simulink library "mylib"  (R2019b)
settings: Solver=VariableStepAuto  StartTime=0.0  StopTime=10.0  RelTol=1e-3
undefined symbols (not defined in the file or in its folder): AG, AH, AV, BCHL, BCHV, BG, BH, CG, CH, magnitude, Ts, XMW
libraries: $bdroot x28, TElib x2
(part 3 of 3)

== system mylib/Process Noise I=1-12 G New/TESUB6/Subsystem/TESUB7(3) ==
  G : Inport
  I : Constant  Value=3
  TESUB7 : $bdroot/TESUB7 G-New  SystemSampleTime=-1  Latency=0  AutoFrameSizeCalculation=off
  TESUB7(3) : Outport  VectorParamsAs1DForOutWhenUnconnected=off
  G_NEW : Outport  Port=2  VectorParamsAs1DForOutWhenUnconnected=off
  wires:
  I/1 -> TESUB7/1
  TESUB7/2 -> G_NEW/1
  G/1 -> TESUB7/2
  TESUB7/1 -> TESUB7(3)/1

== system mylib/Process Noise I=1-12 G New/TESUB6/Subsystem/TESUB7(4) ==
  G : Inport
  I : Constant  Value=4
  TESUB7 : $bdroot/TESUB7 G-New  SystemSampleTime=-1  Latency=0  AutoFrameSizeCalculation=off
  TESUB7(4) : Outport  VectorParamsAs1DForOutWhenUnconnected=off
  G_NEW : Outport  Port=2  VectorParamsAs1DForOutWhenUnconnected=off
  wires:
  I/1 -> TESUB7/1
  TESUB7/2 -> G_NEW/1
  G/1 -> TESUB7/2
  TESUB7/1 -> TESUB7(4)/1

== system mylib/Process Noise I=1-12 G New/TESUB6/Subsystem/TESUB7(5) ==
  G : Inport
  I : Constant  Value=5
  TESUB7 : $bdroot/TESUB7 G-New  SystemSampleTime=-1  Latency=0  AutoFrameSizeCalculation=off
  TESUB7(5) : Outport  VectorParamsAs1DForOutWhenUnconnected=off
  G_NEW : Outport  Port=2  VectorParamsAs1DForOutWhenUnconnected=off
  wires:
  I/1 -> TESUB7/1
  TESUB7/2 -> G_NEW/1
  G/1 -> TESUB7/2
  TESUB7/1 -> TESUB7(5)/1

== system mylib/Process Noise I=1-12 G New/TESUB6/Subsystem/TESUB7(6) ==
  G : Inport
  I : Constant  Value=6
  TESUB7 : $bdroot/TESUB7 G-New  SystemSampleTime=-1  Latency=0  AutoFrameSizeCalculation=off
  TESUB7(6) : Outport  VectorParamsAs1DForOutWhenUnconnected=off
  G_NEW : Outport  Port=2  VectorParamsAs1DForOutWhenUnconnected=off
  wires:
  I/1 -> TESUB7/1
  TESUB7/2 -> G_NEW/1
  G/1 -> TESUB7/2
  TESUB7/1 -> TESUB7(6)/1

== system mylib/Process Noise I=1-12 G New/TESUB6/Subsystem/TESUB7(7) ==
  G : Inport
  I : Constant  Value=7
  TESUB7 : $bdroot/TESUB7 G-New  SystemSampleTime=-1  Latency=0  AutoFrameSizeCalculation=off
  TESUB7(7) : Outport  VectorParamsAs1DForOutWhenUnconnected=off
  G_NEW : Outport  Port=2  VectorParamsAs1DForOutWhenUnconnected=off
  wires:
  I/1 -> TESUB7/1
  TESUB7/2 -> G_NEW/1
  G/1 -> TESUB7/2
  TESUB7/1 -> TESUB7(7)/1

== system mylib/Process Noise I=1-12 G New/TESUB6/Subsystem/TESUB7(8) ==
  G : Inport
  I : Constant  Value=8
  TESUB7 : $bdroot/TESUB7 G-New  SystemSampleTime=-1  Latency=0  AutoFrameSizeCalculation=off
  TESUB7(8) : Outport  VectorParamsAs1DForOutWhenUnconnected=off
  G_NEW : Outport  Port=2  VectorParamsAs1DForOutWhenUnconnected=off
  wires:
  I/1 -> TESUB7/1
  TESUB7/2 -> G_NEW/1
  G/1 -> TESUB7/2
  TESUB7/1 -> TESUB7(8)/1

== system mylib/Process Noise I=1-12 G New/TESUB6/Subsystem/TESUB7(9) ==
  G : Inport
  I : Constant  Value=9
  TESUB7 : $bdroot/TESUB7 G-New  SystemSampleTime=-1  Latency=0  AutoFrameSizeCalculation=off
  TESUB7(9) : Outport  VectorParamsAs1DForOutWhenUnconnected=off
  G_NEW : Outport  Port=2  VectorParamsAs1DForOutWhenUnconnected=off
  wires:
  I/1 -> TESUB7/1
  TESUB7/2 -> G_NEW/1
  G/1 -> TESUB7/2
  TESUB7/1 -> TESUB7(9)/1

== system mylib/Process Noise I=23-36/Gas Analysis Delay/Subsystem/If Action Subsystem ==
  Action Port : ActionPort
  Constant : Constant  Value=0
  Out1 : Outport  VectorParamsAs1DForOutWhenUnconnected=off
  wires:
  Constant/1 -> Out1/1

== system mylib/Process Noise I=23-36/Gas Analysis Delay/Subsystem/If Action Subsystem1 ==
  In1 : Inport
  Action Port : ActionPort
  Out1 : Outport  VectorParamsAs1DForOutWhenUnconnected=off
  wires:
  In1/1 -> Out1/1

== system mylib/Process Noise I=37-41/Gas Analysis Delay/Subsystem/If Action Subsystem ==
  Action Port : ActionPort
  Constant : Constant  Value=0
  Out1 : Outport  VectorParamsAs1DForOutWhenUnconnected=off
  wires:
  Constant/1 -> Out1/1

== system mylib/Process Noise I=37-41/Gas Analysis Delay/Subsystem/If Action Subsystem1 ==
  In1 : Inport
  Action Port : ActionPort
  Out1 : Outport  VectorParamsAs1DForOutWhenUnconnected=off
  wires:
  In1/1 -> Out1/1

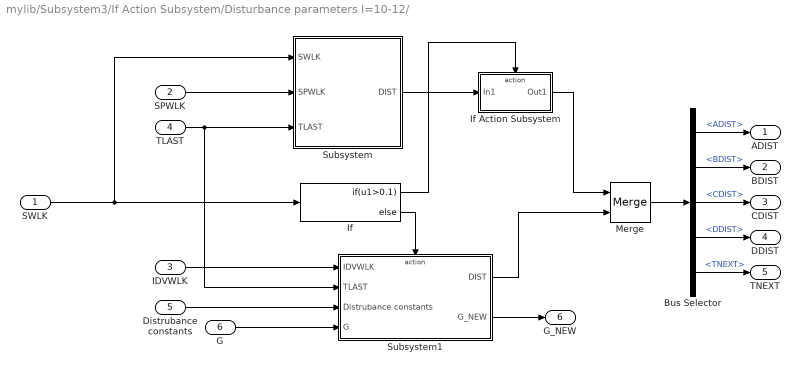
== system mylib/Subsystem3/If Action Subsystem/Disturbance parameters I=10-12/  ==
  SWLK : Inport
  SPWLK : Inport  Port=2
  IDVWLK : Inport  Port=3
  TLAST : Inport  Port=4
  Distrubance constants : Inport  Port=5
  G : Inport  Port=6
  Bus Selector : BusSelector  OutputSignals=ADIST,BDIST,CDIST,DDIST,TNEXT
  If : If  IfExpression=u1>0.1
  If Action Subsystem : Subsystem  TreatAsAtomicUnit=on
  Merge : Merge
  Subsystem : Subsystem
  Subsystem1 : Subsystem
  ADIST : Outport  VectorParamsAs1DForOutWhenUnconnected=off
  BDIST : Outport  Port=2  VectorParamsAs1DForOutWhenUnconnected=off
  CDIST : Outport  Port=3  VectorParamsAs1DForOutWhenUnconnected=off
  DDIST : Outport  Port=4  VectorParamsAs1DForOutWhenUnconnected=off
  TNEXT : Outport  Port=5  VectorParamsAs1DForOutWhenUnconnected=off
  G_NEW : Outport  Port=6  VectorParamsAs1DForOutWhenUnconnected=off
  wires:
  G/1 -> Subsystem1/4(G)
  Bus Selector/5 -> TNEXT/1  "<TNEXT>"
  Bus Selector/4 -> DDIST/1  "<DDIST>"
  Bus Selector/3 -> CDIST/1  "<CDIST>"
  Bus Selector/2 -> BDIST/1  "<BDIST>"
  Bus Selector/1 -> ADIST/1  "<ADIST>"
  Distrubance constants/1 -> Subsystem1/3(Distrubance constants)
  Merge/1 -> Bus Selector/1
  Subsystem1/1(DIST) -> Merge/2
  If Action Subsystem/1(Out1) -> Merge/1
  Subsystem/1(DIST) -> If Action Subsystem/1(In1)
  If/2 -> Subsystem1/Action
  If/1 -> If Action Subsystem/Action
  TLAST/1 -> Subsystem/3(TLAST), Subsystem1/2(TLAST)
  SWLK/1 -> If/1, Subsystem/1(SWLK)
  SPWLK/1 -> Subsystem/2(SPWLK)
  IDVWLK/1 -> Subsystem1/1(IDVWLK)
  Subsystem1/2(G_NEW) -> G_NEW/1

== system mylib/Subsystem3/If Action Subsystem/Disturbance parameters I=10-12/Subsystem ==
  TNEXT : Inport
  TLAST : Inport  Port=2
  HWLK : Sum  Inputs=+-
  "HWLK " : Outport  VectorParamsAs1DForOutWhenUnconnected=off
  wires:
  HWLK/1 -> "HWLK "/1
  TLAST/1 -> HWLK/2
  TNEXT/1 -> HWLK/1

== system mylib/Subsystem3/If Action Subsystem/Disturbance parameters I=10-12/Subsystem1 ==
  ADIST : Inport
  BDIST : Inport  Port=2
  CDIST : Inport  Port=3
  DDIST : Inport  Port=4
  HWLK : Inport  Port=5
  Add : Sum
  Add1 : Sum
  Product : Product
  Product1 : Product
  Product2 : Product
  SWLK : Sum
  "SWLK " : Outport  VectorParamsAs1DForOutWhenUnconnected=off
  wires:
  HWLK/1 -> Product/1, Product1/1, Product2/1
  Add1/1 -> Product2/2
  Product1/1 -> Add1/1
  DDIST/1 -> Product/2
  Product2/1 -> SWLK/2
  Add/1 -> Product1/2
  Product/1 -> Add/1
  SWLK/1 -> "SWLK "/1
  CDIST/1 -> Add/2
  ADIST/1 -> SWLK/1
  BDIST/1 -> Add1/2

== system mylib/Subsystem3/If Action Subsystem/Disturbance parameters I=10-12/Subsystem2 ==
  BDIST : Inport
  CDIST : Inport  Port=2
  DDIST : Inport  Port=3
  HWLK : Inport  Port=4
  Add2 : Sum
  Constant : Constant  Value=3
  Constant1 : Constant  Value=2
  Product3 : Product  Inputs=3
  Product4 : Product
  Product5 : Product
  SPWLK : Sum
  "SPWLK " : Outport  VectorParamsAs1DForOutWhenUnconnected=off
  wires:
  BDIST/1 -> SPWLK/1
  CDIST/1 -> Product4/2
  Constant1/1 -> Product4/1
  Product3/1 -> Add2/1
  HWLK/1 -> Product3/2, Product5/1
  Product5/1 -> SPWLK/2
  Constant/1 -> Product3/1
  Add2/1 -> Product5/2
  SPWLK/1 -> "SPWLK "/1
  Product4/1 -> Add2/2
  DDIST/1 -> Product3/3

== system mylib/Disturbance calculations I=1-9/If Action Subsystem/Disturbance parameters I=1-9/TESUB5/Subsystem ==
  G : Inport
  HSPAN : Inport  Port=2
  HZERO : Inport  Port=3
  Constant : Constant  Value=-1
  H : Sum
  Product : Product
  TESUB7 G-New : $bdroot/TESUB7 G-New  SystemSampleTime=-1  Latency=0  AutoFrameSizeCalculation=off
  "H " : Outport  VectorParamsAs1DForOutWhenUnconnected=off
  G_NEW : Outport  Port=2  VectorParamsAs1DForOutWhenUnconnected=off
  wires:
  HZERO/1 -> H/2
  HSPAN/1 -> Product/1
  Product/1 -> H/1
  H/1 -> "H "/1
  Constant/1 -> TESUB7 G-New/1
  G/1 -> TESUB7 G-New/2
  TESUB7 G-New/1 -> Product/2  "TESUB7"
  TESUB7 G-New/2 -> G_NEW/1

== system mylib/Disturbance calculations I=1-9/If Action Subsystem/Disturbance parameters I=1-9/TESUB5/Subsystem1 ==
  SSPAN : Inport
  G : Inport  Port=2
  SZERO : Inport  Port=3
  IDVFLAG : Inport  Port=4
  Constant : Constant  Value=-1
  Product1 : Product  Inputs=3
  S1 : Sum
  TESUB7 G-New : $bdroot/TESUB7 G-New  SystemSampleTime=-1  Latency=0  AutoFrameSizeCalculation=off
  "S1 " : Outport  VectorParamsAs1DForOutWhenUnconnected=off
  G_NEW : Outport  Port=2  VectorParamsAs1DForOutWhenUnconnected=off
  wires:
  SSPAN/1 -> Product1/1
  IDVFLAG/1 -> Product1/3
  S1/1 -> "S1 "/1
  Product1/1 -> S1/1
  SZERO/1 -> S1/2
  Constant/1 -> TESUB7 G-New/1
  G/1 -> TESUB7 G-New/2
  TESUB7 G-New/1 -> Product1/2  "TESUB7"
  TESUB7 G-New/2 -> G_NEW/1

== system mylib/Disturbance calculations I=1-9/If Action Subsystem/Disturbance parameters I=1-9/TESUB5/Subsystem2 ==
  G : Inport
  SPSPAN : Inport  Port=2
  IDVFLAG : Inport  Port=3
  Constant : Constant  Value=-1
  S1P : Product  Inputs=3
  TESUB7 G-New : $bdroot/TESUB7 G-New  SystemSampleTime=-1  Latency=0  AutoFrameSizeCalculation=off
  "S1P " : Outport  VectorParamsAs1DForOutWhenUnconnected=off
  G_NEW : Outport  Port=2  VectorParamsAs1DForOutWhenUnconnected=off
  wires:
  SPSPAN/1 -> S1P/1
  S1P/1 -> "S1P "/1
  IDVFLAG/1 -> S1P/3
  TESUB7 G-New/1 -> S1P/2  "TESUB7"
  TESUB7 G-New/2 -> G_NEW/1
  Constant/1 -> TESUB7 G-New/1
  G/1 -> TESUB7 G-New/2

== system mylib/Disturbance calculations I=1-9/If Action Subsystem/Disturbance parameters I=1-9/TESUB5/Subsystem3 ==
  SP : Inport
  S1 : Inport  Port=2
  S : Inport  Port=3
  S1P : Inport  Port=4
  H : Inport  Port=5
  Add1 : Sum
  Constant : Constant  Value=3
  Constant1 : Constant  Value=2
  Divide : Product  Inputs=*/
  Math Function : Math  Operator=magnitude^2  SaturateOnIntegerOverflow=on
  Product2 : Product
  Product3 : Product
  Product4 : Product
  Subtract : Sum  Inputs=+-
  Subtract1 : Sum  Inputs=+-
  CDIST : Outport  VectorParamsAs1DForOutWhenUnconnected=off
  wires:
  S1P/1 -> Add1/1
  H/1 -> Math Function/1, Product4/1
  S/1 -> Subtract/2
  Divide/1 -> CDIST/1
  Subtract/1 -> Product2/1
  Add1/1 -> Product4/2
  Constant1/1 -> Product3/2
  SP/1 -> Product3/1
  Constant/1 -> Product2/2
  S1/1 -> Subtract/1
  Product2/1 -> Subtract1/1
  Math Function/1 -> Divide/2
  Product4/1 -> Subtract1/2
  Subtract1/1 -> Divide/1
  Product3/1 -> Add1/2

== system mylib/Disturbance calculations I=1-9/If Action Subsystem/Disturbance parameters I=1-9/TESUB5/Subsystem4 ==
  SP : Inport
  S1 : Inport  Port=2
  S : Inport  Port=3
  S1P : Inport  Port=4
  H : Inport  Port=5
  Add2 : Sum
  Add3 : Sum
  Constant : Constant  Value=3
  Constant1 : Constant  Value=2
  Divide1 : Product  Inputs=*/
  Math Function1 : Math  Operator=pow  SaturateOnIntegerOverflow=on
  Product5 : Product
  Product6 : Product
  Subtract2 : Sum  Inputs=+-
  DDIST : Outport  VectorParamsAs1DForOutWhenUnconnected=off
  wires:
  Constant1/1 -> Product5/2
  S1P/1 -> Add2/1
  S1/1 -> Subtract2/2
  H/1 -> Math Function1/1, Product6/1
  Add3/1 -> Divide1/1
  Constant/1 -> Math Function1/2
  Subtract2/1 -> Product5/1
  Math Function1/1 -> Divide1/2
  Add2/1 -> Product6/2
  S/1 -> Subtract2/1
  Product6/1 -> Add3/2
  SP/1 -> Add2/2
  Divide1/1 -> DDIST/1
  Product5/1 -> Add3/1

== system mylib/Disturbance calculations I=1-9/If Action Subsystem/Disturbance parameters I=1-9/TESUB5/Subsystem5 ==
  TLAST : Inport
  H : Inport  Port=2
  Add : Sum
  TNEXT : Outport  VectorParamsAs1DForOutWhenUnconnected=off
  wires:
  H/1 -> Add/2
  TLAST/1 -> Add/1
  Add/1 -> TNEXT/1

== system mylib/Exergy/Subsystem2/Subsystem1/Entropy of Stream MBtu//lb-mol·°C/If Action Subsystem ==
  In1 : Inport
  Action Port : ActionPort
  Out1 : Outport  VectorParamsAs1DForOutWhenUnconnected=off
  wires:
  In1/1 -> Out1/1

== system mylib/Exergy/Subsystem2/Subsystem1/Entropy of Stream MBtu//lb-mol·°C/If Action Subsystem2 ==
  In1 : Inport
  Action Port : ActionPort
  Out1 : Outport  VectorParamsAs1DForOutWhenUnconnected=off
  wires:
  In1/1 -> Out1/1

== system mylib/Exergy/Subsystem2/Subsystem1/Entropy of Stream MBtu//lb-mol·°C/Molar Liquid Entropy change of stream MBtu//lb-mol·°C ==
  T : Inport
  XST(I,1) : Inport  Port=2
  T0 : Inport  Port=3
  Constant : Constant  Value=XMW
  Product : Product  Inputs=3
  Sum of Elements : Sum  Inputs=+
  s-s0 Entropy change of individual components MBtu/lb·°C : Subsystem
  Cp/T dt : Outport  VectorParamsAs1DForOutWhenUnconnected=off
  wires:
  XST(I,1)/1 -> Product/3
  Constant/1 -> Product/2
  s-s0 Entropy change of individual components MBtu/lb·°C/1("s-s0 MBtu/lb·°C ") -> Product/1
  Product/1 -> Sum of Elements/1
  T/1 -> s-s0 Entropy change of individual components MBtu/lb·°C/1(T)
  Sum of Elements/1 -> Cp/T dt/1
  T0/1 -> s-s0 Entropy change of individual components MBtu/lb·°C/2(T0)

== system mylib/Exergy/Subsystem2/Subsystem1/Entropy of Stream MBtu//lb-mol·°C/Molar Vapour Entropy change of stream MBtu//lb-mol·°C ==
  T : Inport
  XST(I,1) : Inport  Port=2
  T0 : Inport  Port=3
  Constant : Constant  Value=XMW
  Product : Product  Inputs=3
  Sum of Elements : Sum  Inputs=+
  s-s0 Entropy change of individual components MBtu/lb·°C : Subsystem
  Cp/T dt : Outport  VectorParamsAs1DForOutWhenUnconnected=off
  wires:
  XST(I,1)/1 -> Product/3
  s-s0 Entropy change of individual components MBtu/lb·°C/1("s-s0 MBtu/lb·°C ") -> Product/1
  T/1 -> s-s0 Entropy change of individual components MBtu/lb·°C/1(T)
  Constant/1 -> Product/2
  Product/1 -> Sum of Elements/1
  Sum of Elements/1 -> Cp/T dt/1
  T0/1 -> s-s0 Entropy change of individual components MBtu/lb·°C/2(T0)

== system mylib/Exergy Molar Flow/Subsystem2/Subsystem1/Entropy of Stream MBtu//lb-mol·°C/If Action Subsystem ==
  In1 : Inport
  Action Port : ActionPort
  Out1 : Outport  VectorParamsAs1DForOutWhenUnconnected=off
  wires:
  In1/1 -> Out1/1

== system mylib/Exergy Molar Flow/Subsystem2/Subsystem1/Entropy of Stream MBtu//lb-mol·°C/If Action Subsystem2 ==
  In1 : Inport
  Action Port : ActionPort
  Out1 : Outport  VectorParamsAs1DForOutWhenUnconnected=off
  wires:
  In1/1 -> Out1/1

== system mylib/Exergy Molar Flow/Subsystem2/Subsystem1/Entropy of Stream MBtu//lb-mol·°C/Molar Liquid Entropy change of stream MBtu//lb-mol·°C ==
  T : Inport
  XST(I,1) : Inport  Port=2
  T0 : Inport  Port=3
  Constant : Constant  Value=XMW
  Product : Product  Inputs=3
  Sum of Elements : Sum  Inputs=+
  s-s0 Entropy change of individual components MBtu/lb·°C : Subsystem
  Cp/T dt : Outport  VectorParamsAs1DForOutWhenUnconnected=off
  wires:
  T0/1 -> s-s0 Entropy change of individual components MBtu/lb·°C/2(T0)
  Sum of Elements/1 -> Cp/T dt/1
  T/1 -> s-s0 Entropy change of individual components MBtu/lb·°C/1(T)
  Product/1 -> Sum of Elements/1
  s-s0 Entropy change of individual components MBtu/lb·°C/1("s-s0 MBtu/lb·°C ") -> Product/1
  Constant/1 -> Product/2
  XST(I,1)/1 -> Product/3

== system mylib/Exergy Molar Flow/Subsystem2/Subsystem1/Entropy of Stream MBtu//lb-mol·°C/Molar Vapour Entropy change of stream MBtu//lb-mol·°C ==
  T : Inport
  XST(I,1) : Inport  Port=2
  T0 : Inport  Port=3
  Constant : Constant  Value=XMW
  Product : Product  Inputs=3
  Sum of Elements : Sum  Inputs=+
  s-s0 Entropy change of individual components MBtu/lb·°C : Subsystem
  Cp/T dt : Outport  VectorParamsAs1DForOutWhenUnconnected=off
  wires:
  T0/1 -> s-s0 Entropy change of individual components MBtu/lb·°C/2(T0)
  Sum of Elements/1 -> Cp/T dt/1
  Product/1 -> Sum of Elements/1
  Constant/1 -> Product/2
  T/1 -> s-s0 Entropy change of individual components MBtu/lb·°C/1(T)
  s-s0 Entropy change of individual components MBtu/lb·°C/1("s-s0 MBtu/lb·°C ") -> Product/1
  XST(I,1)/1 -> Product/3

== system mylib/Subsystem3/If Action Subsystem/Disturbance parameters I=10-12/ /If Action Subsystem ==
  In1 : Inport
  Action Port : ActionPort
  Out1 : Outport  VectorParamsAs1DForOutWhenUnconnected=off
  wires:
  In1/1 -> Out1/1

== system mylib/Subsystem3/If Action Subsystem/Disturbance parameters I=10-12/ /Subsystem ==
  SWLK : Inport
  SPWLK : Inport  Port=2
  TLAST : Inport  Port=3
  ADIST : Gain
  Add : Sum
  BDIST : Gain
  Bus Creator : BusCreator  Inputs=5
  Constant : Constant  Value=0.1
  Subsystem : Subsystem
  Subsystem1 : Subsystem
  DIST : Outport  VectorParamsAs1DForOutWhenUnconnected=off
  wires:
  Bus Creator/1 -> DIST/1
  Add/1 -> Bus Creator/5  "TNEXT"
  Constant/1 -> Add/2
  TLAST/1 -> Add/1
  Subsystem1/1(DDIST) -> Bus Creator/4  "DDIST"
  Subsystem/1(CDIST) -> Bus Creator/3  "CDIST"
  BDIST/1 -> Bus Creator/2  "BDIST"
  ADIST/1 -> Bus Creator/1  "ADIST"
  SPWLK/1 -> BDIST/1, Subsystem/2(SPWLK), Subsystem1/2(SPWLK)
  SWLK/1 -> ADIST/1, Subsystem/1(SWLK), Subsystem1/1(SWLK)

== system mylib/Subsystem3/If Action Subsystem/Disturbance parameters I=10-12/ /Subsystem1 ==
  IDVWLK : Inport
  TLAST : Inport  Port=2
  Distrubance constants : Inport  Port=3
  G : Inport  Port=4
  Action Port : ActionPort
  Add : Sum
  Bus Creator : BusCreator  Inputs=5
  Constant : Constant  Value=0.0
  Constant1 : Constant  Value=0.0
  Constant2 : Constant  Value=0.0
  Divide : Product  Inputs=*/
  HWLK : Subsystem
  Math Function : Math  Operator=magnitude^2  SaturateOnIntegerOverflow=on
  DIST : Outport  VectorParamsAs1DForOutWhenUnconnected=off
  G_NEW : Outport  Port=2  OutputWhenDisabled=reset  InitialOutput=0  VectorParamsAs1DForOutWhenUnconnected=off
  wires:
  G/1 -> HWLK/2(G)
  IDVWLK/1 -> Divide/1
  Divide/1 -> Bus Creator/3  "CDIST"
  Math Function/1 -> Divide/2
  Add/1 -> Bus Creator/5  "TNEXT"
  HWLK/1(HWLK) -> Math Function/1, Add/2
  TLAST/1 -> Add/1
  Distrubance constants/1 -> HWLK/1(Distrubance constants)
  Constant2/1 -> Bus Creator/4  "DDIST"
  Constant1/1 -> Bus Creator/2  "BDIST"
  Constant/1 -> Bus Creator/1  "ADIST"
  Bus Creator/1 -> DIST/1
  HWLK/2(G_NEW) -> G_NEW/1

== system mylib/Exergy/Subsystem2/Subsystem1/Entropy of Stream MBtu//lb-mol·°C/Molar Liquid Entropy change of stream MBtu//lb-mol·°C/s-s0 Entropy change of individual components MBtu//lb·°C ==
  T : Inport
  T0 : Inport  Port=2
  "     " : Product
  Add : Sum  Inputs=3
  MBtu/lb·°F : Subsystem
      mask Display: disp('Aln(T/T0)', 'texmode', 'on')
  "MBtu/lb·°F " : Subsystem
      mask Display: disp('B(T-T0)', 'texmode', 'on')
  "MBtu/lb·°F   " : Subsystem
      mask Display: disp('(C/2)*(T^2-T0^2)', 'texmode', 'on')
  To convert °F to °C : Constant  Value=1.8
  "s-s0 MBtu/lb·°C " : Outport  VectorParamsAs1DForOutWhenUnconnected=off
  wires:
  "MBtu/lb·°F "/1(Out1) -> Add/2
  "     "/1 -> "s-s0 MBtu/lb·°C "/1
  MBtu/lb·°F/1(Out1) -> Add/1
  To convert °F to °C/1 -> "     "/2
  "MBtu/lb·°F   "/1(Out1) -> Add/3
  T/1 -> "MBtu/lb·°F   "/1(T), "MBtu/lb·°F "/1(T), MBtu/lb·°F/1(T)
  T0/1 -> "MBtu/lb·°F   "/2(T0), "MBtu/lb·°F "/2(T0), MBtu/lb·°F/2(T0)
  Add/1 -> "     "/1

== system mylib/Exergy/Subsystem2/Subsystem1/Entropy of Stream MBtu//lb-mol·°C/Molar Vapour Entropy change of stream MBtu//lb-mol·°C/s-s0 Entropy change of individual components MBtu//lb·°C ==
  T : Inport
  T0 : Inport  Port=2
  "     " : Product
  Add : Sum  Inputs=3
  MBtu/lb·°F : Subsystem
      mask Display: disp('Aln(T/T0)', 'texmode', 'on')
  "MBtu/lb·°F " : Subsystem
      mask Display: disp('B(T-T0)', 'texmode', 'on')
  "MBtu/lb·°F   " : Subsystem
      mask Display: disp('(C/2)*(T^2-T0^2)', 'texmode', 'on')
  To convert °F to °C : Constant  Value=1.8
  "s-s0 MBtu/lb·°C " : Outport  VectorParamsAs1DForOutWhenUnconnected=off
  wires:
  "MBtu/lb·°F "/1(Out1) -> Add/2
  "     "/1 -> "s-s0 MBtu/lb·°C "/1
  MBtu/lb·°F/1(Out1) -> Add/1
  To convert °F to °C/1 -> "     "/2
  "MBtu/lb·°F   "/1(Out1) -> Add/3
  T/1 -> "MBtu/lb·°F   "/1(T), "MBtu/lb·°F "/1(T), MBtu/lb·°F/1(T)
  T0/1 -> "MBtu/lb·°F   "/2(T0), "MBtu/lb·°F "/2(T0), MBtu/lb·°F/2(T0)
  Add/1 -> "     "/1

== system mylib/Exergy Molar Flow/Subsystem2/Subsystem1/Entropy of Stream MBtu//lb-mol·°C/Molar Liquid Entropy change of stream MBtu//lb-mol·°C/s-s0 Entropy change of individual components MBtu//lb·°C ==
  T : Inport
  T0 : Inport  Port=2
  "     " : Product
  Add : Sum  Inputs=3
  MBtu/lb·°F : Subsystem
      mask Display: disp('Aln(T/T0)', 'texmode', 'on')
  "MBtu/lb·°F " : Subsystem
      mask Display: disp('B(T-T0)', 'texmode', 'on')
  "MBtu/lb·°F   " : Subsystem
      mask Display: disp('(C/2)*(T^2-T0^2)', 'texmode', 'on')
  To convert °F to °C : Constant  Value=1.8
  "s-s0 MBtu/lb·°C " : Outport  VectorParamsAs1DForOutWhenUnconnected=off
  wires:
  Add/1 -> "     "/1
  T0/1 -> MBtu/lb·°F/2(T0), "MBtu/lb·°F "/2(T0), "MBtu/lb·°F   "/2(T0)
  T/1 -> MBtu/lb·°F/1(T), "MBtu/lb·°F "/1(T), "MBtu/lb·°F   "/1(T)
  "MBtu/lb·°F   "/1(Out1) -> Add/3
  To convert °F to °C/1 -> "     "/2
  MBtu/lb·°F/1(Out1) -> Add/1
  "     "/1 -> "s-s0 MBtu/lb·°C "/1
  "MBtu/lb·°F "/1(Out1) -> Add/2

== system mylib/Exergy Molar Flow/Subsystem2/Subsystem1/Entropy of Stream MBtu//lb-mol·°C/Molar Vapour Entropy change of stream MBtu//lb-mol·°C/s-s0 Entropy change of individual components MBtu//lb·°C ==
  T : Inport
  T0 : Inport  Port=2
  "     " : Product
  Add : Sum  Inputs=3
  MBtu/lb·°F : Subsystem
      mask Display: disp('Aln(T/T0)', 'texmode', 'on')
  "MBtu/lb·°F " : Subsystem
      mask Display: disp('B(T-T0)', 'texmode', 'on')
  "MBtu/lb·°F   " : Subsystem
      mask Display: disp('(C/2)*(T^2-T0^2)', 'texmode', 'on')
  To convert °F to °C : Constant  Value=1.8
  "s-s0 MBtu/lb·°C " : Outport  VectorParamsAs1DForOutWhenUnconnected=off
  wires:
  Add/1 -> "     "/1
  T0/1 -> MBtu/lb·°F/2(T0), "MBtu/lb·°F "/2(T0), "MBtu/lb·°F   "/2(T0)
  T/1 -> MBtu/lb·°F/1(T), "MBtu/lb·°F "/1(T), "MBtu/lb·°F   "/1(T)
  "MBtu/lb·°F   "/1(Out1) -> Add/3
  To convert °F to °C/1 -> "     "/2
  MBtu/lb·°F/1(Out1) -> Add/1
  "     "/1 -> "s-s0 MBtu/lb·°C "/1
  "MBtu/lb·°F "/1(Out1) -> Add/2

== system mylib/Subsystem3/If Action Subsystem/Disturbance parameters I=10-12/ /Subsystem/Subsystem ==
  SWLK : Inport
  SPWLK : Inport  Port=2
  Add : Sum
  Constant : Constant  Value=3
  Constant1 : Constant  Value=0.2
  Constant2 : Constant  Value=0.01
  Divide : Product  Inputs=*/
  Product : Product
  Product1 : Product
  Unary Minus : UnaryMinus
  CDIST : Outport  VectorParamsAs1DForOutWhenUnconnected=off
  wires:
  Divide/1 -> CDIST/1
  Constant2/1 -> Divide/2
  Unary Minus/1 -> Divide/1
  Add/1 -> Unary Minus/1
  Product1/1 -> Add/2
  Product/1 -> Add/1
  SPWLK/1 -> Product1/2
  SWLK/1 -> Product/2
  Constant1/1 -> Product1/1
  Constant/1 -> Product/1

== system mylib/Subsystem3/If Action Subsystem/Disturbance parameters I=10-12/ /Subsystem/Subsystem1 ==
  SWLK : Inport
  SPWLK : Inport  Port=2
  Add : Sum
  Constant : Constant  Value=2
  Constant1 : Constant  Value=0.1
  Constant2 : Constant  Value=0.001
  Divide : Product  Inputs=*/
  Product : Product
  Product1 : Product
  DDIST : Outport  VectorParamsAs1DForOutWhenUnconnected=off
  wires:
  Divide/1 -> DDIST/1
  Constant2/1 -> Divide/2
  Add/1 -> Divide/1
  Product1/1 -> Add/2
  Product/1 -> Add/1
  SPWLK/1 -> Product1/2
  SWLK/1 -> Product/2
  Constant1/1 -> Product1/1
  Constant/1 -> Product/1

== system mylib/Subsystem3/If Action Subsystem/Disturbance parameters I=10-12/ /Subsystem1/HWLK ==
  Distrubance constants : Inport
  G : Inport  Port=2
  Add : Sum
  Bus Selector : BusSelector  OutputSignals=HSPAN,HZERO
  Constant : Constant  Value=-1
  Product : Product
  TESUB7 G-New : $bdroot/TESUB7 G-New  SystemSampleTime=-1  Latency=0  AutoFrameSizeCalculation=off
  HWLK : Outport  VectorParamsAs1DForOutWhenUnconnected=off
  G_NEW : Outport  Port=2  OutputWhenDisabled=reset  InitialOutput=[0]  VectorParamsAs1DForOutWhenUnconnected=off
  wires:
  Add/1 -> HWLK/1
  Bus Selector/2 -> Add/2  "<HZERO>"
  Product/1 -> Add/1
  Bus Selector/1 -> Product/2  "<HSPAN>"
  TESUB7 G-New/1 -> Product/1
  Distrubance constants/1 -> Bus Selector/1
  Constant/1 -> TESUB7 G-New/1
  G/1 -> TESUB7 G-New/2
  TESUB7 G-New/2 -> G_NEW/1

== system mylib/Exergy/Subsystem2/Subsystem1/Entropy of Stream MBtu//lb-mol·°C/Molar Liquid Entropy change of stream MBtu//lb-mol·°C/s-s0 Entropy change of individual components MBtu//lb·°C/MBtu//lb·°F ==
  T : Inport
  T0 : Inport  Port=2
  "         " : Product  Inputs=**
  "AH(I) Coefficient A to determine Enthalpy MBtu/lb·°F " : Constant  Value=AH
  Divide : Product  Inputs=*/
  Math Function : Math  Operator=log  SaturateOnIntegerOverflow=on
  Out1 : Outport  VectorParamsAs1DForOutWhenUnconnected=off
  wires:
  "         "/1 -> Out1/1
  "AH(I) Coefficient A to determine Enthalpy MBtu/lb·°F "/1 -> "         "/1
  T0/1 -> Divide/2
  T/1 -> Divide/1
  Math Function/1 -> "         "/2
  Divide/1 -> Math Function/1

== system mylib/Exergy/Subsystem2/Subsystem1/Entropy of Stream MBtu//lb-mol·°C/Molar Liquid Entropy change of stream MBtu//lb-mol·°C/s-s0 Entropy change of individual components MBtu//lb·°C/MBtu//lb·°F  ==
  T : Inport
  T0 : Inport  Port=2
  "         " : Product  Inputs=**
  BH(I) Coefficient B to determine Enthalpy MBtu/lb·°F² : Constant  Value=BH
  Subtract : Sum  Inputs=+-
  Out1 : Outport  VectorParamsAs1DForOutWhenUnconnected=off
  wires:
  "         "/1 -> Out1/1
  BH(I) Coefficient B to determine Enthalpy MBtu/lb·°F²/1 -> "         "/1
  T/1 -> Subtract/1
  T0/1 -> Subtract/2
  Subtract/1 -> "         "/2

== system mylib/Exergy/Subsystem2/Subsystem1/Entropy of Stream MBtu//lb-mol·°C/Molar Liquid Entropy change of stream MBtu//lb-mol·°C/s-s0 Entropy change of individual components MBtu//lb·°C/MBtu//lb·°F    ==
  T : Inport
  T0 : Inport  Port=2
  "        " : Product  Inputs=**
  CH(I) Coefficient C to determine Enthalpy MBtu/lb·°F³ : Constant  Value=CH
  Constant : Constant  Value=2
  Divide : Product  Inputs=*/
  Math Function : Math  Operator=magnitude^2  SaturateOnIntegerOverflow=on
  Math Function1 : Math  Operator=magnitude^2  SaturateOnIntegerOverflow=on
  Subtract : Sum  Inputs=+-
  Out1 : Outport  VectorParamsAs1DForOutWhenUnconnected=off
  wires:
  T/1 -> Math Function/1
  "        "/1 -> Out1/1
  CH(I) Coefficient C to determine Enthalpy MBtu/lb·°F³/1 -> Divide/1
  Constant/1 -> Divide/2
  Divide/1 -> "        "/1
  T0/1 -> Math Function1/1
  Math Function/1 -> Subtract/1
  Math Function1/1 -> Subtract/2
  Subtract/1 -> "        "/2

== system mylib/Exergy/Subsystem2/Subsystem1/Entropy of Stream MBtu//lb-mol·°C/Molar Vapour Entropy change of stream MBtu//lb-mol·°C/s-s0 Entropy change of individual components MBtu//lb·°C/MBtu//lb·°F ==
  T : Inport
  T0 : Inport  Port=2
  "         " : Product  Inputs=**
  "AG(I) Coefficient A to determine Enthalpy MBtu/lb·°F " : Constant  Value=AG
  Divide : Product  Inputs=*/
  Math Function : Math  Operator=log  SaturateOnIntegerOverflow=on
  Out1 : Outport  VectorParamsAs1DForOutWhenUnconnected=off
  wires:
  "         "/1 -> Out1/1
  "AG(I) Coefficient A to determine Enthalpy MBtu/lb·°F "/1 -> "         "/1
  T0/1 -> Divide/2
  T/1 -> Divide/1
  Math Function/1 -> "         "/2
  Divide/1 -> Math Function/1

== system mylib/Exergy/Subsystem2/Subsystem1/Entropy of Stream MBtu//lb-mol·°C/Molar Vapour Entropy change of stream MBtu//lb-mol·°C/s-s0 Entropy change of individual components MBtu//lb·°C/MBtu//lb·°F  ==
  T : Inport
  T0 : Inport  Port=2
  "         " : Product  Inputs=**
  BH(I) Coefficient B to determine Enthalpy MBtu/lb·°F²1 : Constant  Value=BG
  Subtract : Sum  Inputs=+-
  Out1 : Outport  VectorParamsAs1DForOutWhenUnconnected=off
  wires:
  "         "/1 -> Out1/1
  BH(I) Coefficient B to determine Enthalpy MBtu/lb·°F²1/1 -> "         "/1
  T/1 -> Subtract/1
  T0/1 -> Subtract/2
  Subtract/1 -> "         "/2

== system mylib/Exergy/Subsystem2/Subsystem1/Entropy of Stream MBtu//lb-mol·°C/Molar Vapour Entropy change of stream MBtu//lb-mol·°C/s-s0 Entropy change of individual components MBtu//lb·°C/MBtu//lb·°F    ==
  T : Inport
  T0 : Inport  Port=2
  "        " : Product  Inputs=**
  CH(I) Coefficient C to determine Enthalpy MBtu/lb·°F³ : Constant  Value=CG
  Constant : Constant  Value=2
  Divide : Product  Inputs=*/
  Math Function : Math  Operator=magnitude^2  SaturateOnIntegerOverflow=on
  Math Function1 : Math  Operator=magnitude^2  SaturateOnIntegerOverflow=on
  Subtract : Sum  Inputs=+-
  Out1 : Outport  VectorParamsAs1DForOutWhenUnconnected=off
  wires:
  T/1 -> Math Function/1
  "        "/1 -> Out1/1
  CH(I) Coefficient C to determine Enthalpy MBtu/lb·°F³/1 -> Divide/1
  Constant/1 -> Divide/2
  Divide/1 -> "        "/1
  T0/1 -> Math Function1/1
  Math Function/1 -> Subtract/1
  Math Function1/1 -> Subtract/2
  Subtract/1 -> "        "/2

== system mylib/Exergy Molar Flow/Subsystem2/Subsystem1/Entropy of Stream MBtu//lb-mol·°C/Molar Liquid Entropy change of stream MBtu//lb-mol·°C/s-s0 Entropy change of individual components MBtu//lb·°C/MBtu//lb·°F ==
  T : Inport
  T0 : Inport  Port=2
  "         " : Product  Inputs=**
  "AH(I) Coefficient A to determine Enthalpy MBtu/lb·°F " : Constant  Value=AH
  Divide : Product  Inputs=*/
  Math Function : Math  Operator=log  SaturateOnIntegerOverflow=on
  Out1 : Outport  VectorParamsAs1DForOutWhenUnconnected=off
  wires:
  Divide/1 -> Math Function/1
  Math Function/1 -> "         "/2
  T/1 -> Divide/1
  T0/1 -> Divide/2
  "AH(I) Coefficient A to determine Enthalpy MBtu/lb·°F "/1 -> "         "/1
  "         "/1 -> Out1/1

== system mylib/Exergy Molar Flow/Subsystem2/Subsystem1/Entropy of Stream MBtu//lb-mol·°C/Molar Liquid Entropy change of stream MBtu//lb-mol·°C/s-s0 Entropy change of individual components MBtu//lb·°C/MBtu//lb·°F  ==
  T : Inport
  T0 : Inport  Port=2
  "         " : Product  Inputs=**
  BH(I) Coefficient B to determine Enthalpy MBtu/lb·°F² : Constant  Value=BH
  Subtract : Sum  Inputs=+-
  Out1 : Outport  VectorParamsAs1DForOutWhenUnconnected=off
  wires:
  Subtract/1 -> "         "/2
  T0/1 -> Subtract/2
  T/1 -> Subtract/1
  BH(I) Coefficient B to determine Enthalpy MBtu/lb·°F²/1 -> "         "/1
  "         "/1 -> Out1/1

== system mylib/Exergy Molar Flow/Subsystem2/Subsystem1/Entropy of Stream MBtu//lb-mol·°C/Molar Liquid Entropy change of stream MBtu//lb-mol·°C/s-s0 Entropy change of individual components MBtu//lb·°C/MBtu//lb·°F    ==
  T : Inport
  T0 : Inport  Port=2
  "        " : Product  Inputs=**
  CH(I) Coefficient C to determine Enthalpy MBtu/lb·°F³ : Constant  Value=CH
  Constant : Constant  Value=2
  Divide : Product  Inputs=*/
  Math Function : Math  Operator=magnitude^2  SaturateOnIntegerOverflow=on
  Math Function1 : Math  Operator=magnitude^2  SaturateOnIntegerOverflow=on
  Subtract : Sum  Inputs=+-
  Out1 : Outport  VectorParamsAs1DForOutWhenUnconnected=off
  wires:
  Subtract/1 -> "        "/2
  Math Function1/1 -> Subtract/2
  Math Function/1 -> Subtract/1
  T0/1 -> Math Function1/1
  Divide/1 -> "        "/1
  Constant/1 -> Divide/2
  CH(I) Coefficient C to determine Enthalpy MBtu/lb·°F³/1 -> Divide/1
  "        "/1 -> Out1/1
  T/1 -> Math Function/1

== system mylib/Exergy Molar Flow/Subsystem2/Subsystem1/Entropy of Stream MBtu//lb-mol·°C/Molar Vapour Entropy change of stream MBtu//lb-mol·°C/s-s0 Entropy change of individual components MBtu//lb·°C/MBtu//lb·°F ==
  T : Inport
  T0 : Inport  Port=2
  "         " : Product  Inputs=**
  "AG(I) Coefficient A to determine Enthalpy MBtu/lb·°F " : Constant  Value=AG
  Divide : Product  Inputs=*/
  Math Function : Math  Operator=log  SaturateOnIntegerOverflow=on
  Out1 : Outport  VectorParamsAs1DForOutWhenUnconnected=off
  wires:
  Divide/1 -> Math Function/1
  Math Function/1 -> "         "/2
  T/1 -> Divide/1
  T0/1 -> Divide/2
  "AG(I) Coefficient A to determine Enthalpy MBtu/lb·°F "/1 -> "         "/1
  "         "/1 -> Out1/1

== system mylib/Exergy Molar Flow/Subsystem2/Subsystem1/Entropy of Stream MBtu//lb-mol·°C/Molar Vapour Entropy change of stream MBtu//lb-mol·°C/s-s0 Entropy change of individual components MBtu//lb·°C/MBtu//lb·°F  ==
  T : Inport
  T0 : Inport  Port=2
  "         " : Product  Inputs=**
  BH(I) Coefficient B to determine Enthalpy MBtu/lb·°F²1 : Constant  Value=BG
  Subtract : Sum  Inputs=+-
  Out1 : Outport  VectorParamsAs1DForOutWhenUnconnected=off
  wires:
  Subtract/1 -> "         "/2
  T0/1 -> Subtract/2
  T/1 -> Subtract/1
  BH(I) Coefficient B to determine Enthalpy MBtu/lb·°F²1/1 -> "         "/1
  "         "/1 -> Out1/1

== system mylib/Exergy Molar Flow/Subsystem2/Subsystem1/Entropy of Stream MBtu//lb-mol·°C/Molar Vapour Entropy change of stream MBtu//lb-mol·°C/s-s0 Entropy change of individual components MBtu//lb·°C/MBtu//lb·°F    ==
  T : Inport
  T0 : Inport  Port=2
  "        " : Product  Inputs=**
  CH(I) Coefficient C to determine Enthalpy MBtu/lb·°F³ : Constant  Value=CG
  Constant : Constant  Value=2
  Divide : Product  Inputs=*/
  Math Function : Math  Operator=magnitude^2  SaturateOnIntegerOverflow=on
  Math Function1 : Math  Operator=magnitude^2  SaturateOnIntegerOverflow=on
  Subtract : Sum  Inputs=+-
  Out1 : Outport  VectorParamsAs1DForOutWhenUnconnected=off
  wires:
  Subtract/1 -> "        "/2
  Math Function1/1 -> Subtract/2
  Math Function/1 -> Subtract/1
  T0/1 -> Math Function1/1
  Divide/1 -> "        "/1
  Constant/1 -> Divide/2
  CH(I) Coefficient C to determine Enthalpy MBtu/lb·°F³/1 -> Divide/1
  "        "/1 -> Out1/1
  T/1 -> Math Function/1
